simulink library "honestlibrary"  (R2013b)
settings: Solver=ode45  StartTime=0.0  StopTime=10.0  RelTol=1e-3
libraries: honestlibrary x192, xbsIndex_r4 x32
(part 1 of 2)
settings Model: Creator=sergio  LastModifiedBy=root

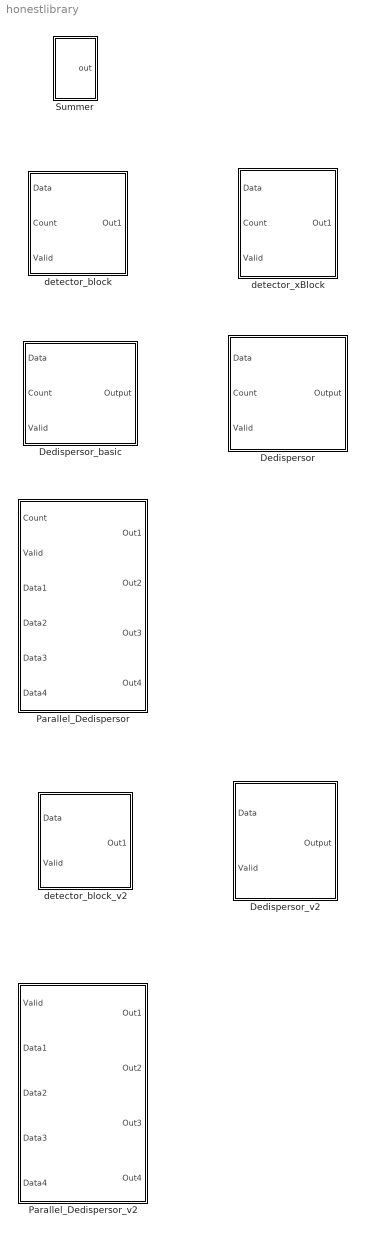
== system honestlibrary ==
  Dedispersor : Subsystem  mask(Detector de FRB (hasta 1024 canales)){DM_Vector=[0:1:15]}
      mask prompts: DM_Vector "DM Vector"
      mask help: Recibe un vector de DM asociado al retardo de cada canal y genera bloques detectores básicos para dedispersar la señal entregada.
      mask init:
      | config.source = str2func('honest_detectorv2');
      | config.toplevel = gcb;
      | config.depend = {'honest_detectorv2.m'};
      | xBlock(config, {DM_Vector});
  Dedispersor_basic : Subsystem  mask(Detector de FRB (hasta 31 canales)){DM_Vector=[0:1:31]}
      mask prompts: DM_Vector "DM Vector"
      mask help: Recibe un vector de DM asociado al retardo de cada canal y genera bloques detectores básicos para dedispersar la señal entregada.
      mask init:
      | config.source = str2func('honest_detector');
      | config.toplevel = gcb;
      | config.depend = {'honest_detector.m'};
      | xBlock(config, {DM_Vector});
  Dedispersor_v2 : Subsystem  mask(Detector de FRB (hasta 1024 canales)){DM_Vector=[0:1:15]}
      mask prompts: DM_Vector "DM Vector"
      mask help:
      | Recibe un vector de DM asociado al retardo de cada canal y genera bloques detectores básicos para dedispersar la señal entregada.
      | Esta versión incorpora un contador de nbits en cada bloque de dedispersión.
      mask init:
      | config.source = str2func('honest_detector_v2');
      | config.toplevel = gcb;
      | config.depend = {'honest_detector_v2.m'};
      | xBlock(config, {DM_Vector});
  Parallel_Dedispersor : Subsystem  mask(Parallel Dedispersor){n_inputs=4, DM_Vector=[1:1:64]}
      mask prompts: n_inputs "Number of Inputs"; DM_Vector "DM Vector"
      mask help:
      | Parallel dedispersor takes two parameters:
      |
      | - DM Vector
      | - Number of Inputs
      |
      | Then dedisperses the incoming serial or n-bus channels according to the DM Vector format. Each input can handle 1023 different channels.
      mask init:
      | honest_parallel_detector_init(gcb,'n_inputs',n_inputs,'DM_Vector',DM_Vector);
      settings: AttributesFormatString=Inputs: 4, Channels: 64
  Parallel_Dedispersor_v2 : Subsystem  mask(Parallel Dedispersor v2){DM_Vector=[1:1:64], n_inputs=4}
      mask prompts: DM_Vector "DM Vector"; n_inputs "Number of Inputs"
      mask help:
      | Parallel dedispersor (v2) takes three parameters:
      |
      | - DM Vector
      | - Number of Inputs
      | - Number of Bits (Counter)
      |
      | Then dedisperses the incoming serial or n-bus channels according to the DM Vector format. Each input can handle 1023 different channels.
      | Each detector block contains a counter activated by the valid signal.
      mask init:
      | honest_parallel_detector_init_v2(gcb,'n_inputs',n_inputs,'DM_Vector',DM_Vector)
      settings: AttributesFormatString=Inputs: 4, Channels: 64
  Summer : Subsystem  mask(summer){num1=1, num2=1}
      mask prompts: num1 "Number 1"; num2 "Number 2"
      mask help: It adds things
      mask init:
      | summer_init(gcb,'num1',num1,'num2',num2);
      settings: AttributesFormatString=1,1
      mask Help: (you can add HTML here to make ir more beauty)
  detector_block : Subsystem  mask(Basic block for FRB detection){chn=3, lat=3}
      mask prompts: chn "Channel"; lat "Latency"
      mask help: Delays a certain channel a number of latency clock cycles, according to the fixed DM table.
      mask init:
      | detector_block_init(gcb,'chn',chn,'lat',lat)
      settings: AttributesFormatString=3,3
      mask Display:
      | port_label ('input',1,'Data')
      | port_label ('input',2,'Count')
      | port_label ('input',3,'En')
      | port_label ('output',1,'Out')
  detector_block_v2 : Subsystem  mask(Basic block for FRB detection){chn=4, lat=9, nbits=2}
      mask prompts: chn "Channel"; lat "Latency"; nbits "Number of Bits (Counter)"
      mask help:
      | Delays a certain channel a number of latency clock cycles, according to the fixed DM table.
      | This version incorporates an internal counter (nbits) to know when store or give a certain value.
      mask init:
      | detector_block_init_v2(gcb,'chn',chn,'lat',lat,'nbits',nbits)
      settings: AttributesFormatString=Channel: 4, Delay: 9
  detector_xBlock : Subsystem  RequirementInfo="{}  %GIDa_91708f24_1105_4a04_a381_067cf6e93763"  mask(Basic block for FRB detection){channel=2, latency=9}
      mask prompts: channel "Channel Number"
      mask help: Delays a certain channel a number of latency clock cycles, according to a fixed DM table.
      mask init:
      | config.source = str2func('detector_xblock');
      | config.toplevel = gcb;
      | config.depend = {'detector_xblock.m'};
      | xBlock(config, {channel, latency});
      | set_param(gcb, 'AttributesFormatString',[num2str(channel),',',num2str(latency)])
      settings: AttributesFormatString=2,9

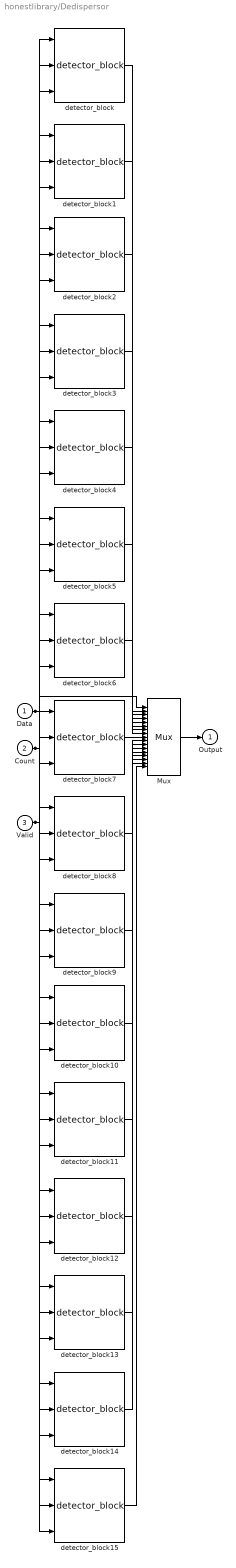
== system honestlibrary/Dedispersor ==
  Data : Inport
  Count : Inport  Port=2
  Valid : Inport  Port=3
  Mux : xbsIndex_r4/Mux  inputs=16  en=off  latency=0  precision=Full  arith_type=Unsigned  n_bits=16  bin_pt=14  quantization=Truncate  overflow=Wrap  dbl_ovrd=off  block_type=mux
  detector_block : honestlibrary/detector_block  chn=0  lat=1
      settings: AttributesFormatString=3,3
  detector_block1 : honestlibrary/detector_block  chn=1  lat=2
      settings: AttributesFormatString=3,3
  detector_block10 : honestlibrary/detector_block  chn=10  lat=11
      settings: AttributesFormatString=3,3
  detector_block11 : honestlibrary/detector_block  chn=11  lat=12
      settings: AttributesFormatString=3,3
  detector_block12 : honestlibrary/detector_block  chn=12  lat=13
      settings: AttributesFormatString=3,3
  detector_block13 : honestlibrary/detector_block  chn=13  lat=14
      settings: AttributesFormatString=3,3
  detector_block14 : honestlibrary/detector_block  chn=14  lat=15
      settings: AttributesFormatString=3,3
  detector_block15 : honestlibrary/detector_block  chn=15  lat=16
      settings: AttributesFormatString=3,3
  detector_block2 : honestlibrary/detector_block  chn=2  lat=3
      settings: AttributesFormatString=3,3
  detector_block3 : honestlibrary/detector_block  chn=3  lat=4
      settings: AttributesFormatString=3,3
  detector_block4 : honestlibrary/detector_block  chn=4  lat=5
      settings: AttributesFormatString=3,3
  detector_block5 : honestlibrary/detector_block  chn=5  lat=6
      settings: AttributesFormatString=3,3
  detector_block6 : honestlibrary/detector_block  chn=6  lat=7
      settings: AttributesFormatString=3,3
  detector_block7 : honestlibrary/detector_block  chn=7  lat=8
      settings: AttributesFormatString=3,3
  detector_block8 : honestlibrary/detector_block  chn=8  lat=9
      settings: AttributesFormatString=3,3
  detector_block9 : honestlibrary/detector_block  chn=9  lat=10
      settings: AttributesFormatString=3,3
  Output : Outport
  wires:
  Data/1 -> detector_block15/1, detector_block14/1, detector_block13/1, detector_block12/1, detector_block11/1, detector_block10/1, detector_block9/1, detector_block8/1, detector_block7/1, detector_block6/1, detector_block5/1, detector_block4/1, detector_block3/1, detector_block2/1, detector_block1/1, detector_block/1
  Count/1 -> Mux/1, detector_block15/2, detector_block14/2, detector_block13/2, detector_block12/2, detector_block11/2, detector_block10/2, detector_block9/2, detector_block8/2, detector_block7/2, detector_block6/2, detector_block5/2, detector_block4/2, detector_block3/2, detector_block2/2, detector_block1/2, detector_block/2
  Valid/1 -> detector_block15/3, detector_block14/3, detector_block13/3, detector_block12/3, detector_block11/3, detector_block10/3, detector_block9/3, detector_block8/3, detector_block7/3, detector_block6/3, detector_block5/3, detector_block4/3, detector_block3/3, detector_block2/3, detector_block1/3, detector_block/3
  Mux/1 -> Output/1
  detector_block15/1 -> Mux/17
  detector_block14/1 -> Mux/16
  detector_block13/1 -> Mux/15
  detector_block12/1 -> Mux/14
  detector_block11/1 -> Mux/13
  detector_block10/1 -> Mux/12
  detector_block9/1 -> Mux/11
  detector_block8/1 -> Mux/10
  detector_block7/1 -> Mux/9
  detector_block6/1 -> Mux/8
  detector_block5/1 -> Mux/7
  detector_block4/1 -> Mux/6
  detector_block3/1 -> Mux/5
  detector_block2/1 -> Mux/4
  detector_block1/1 -> Mux/3
  detector_block/1 -> Mux/2

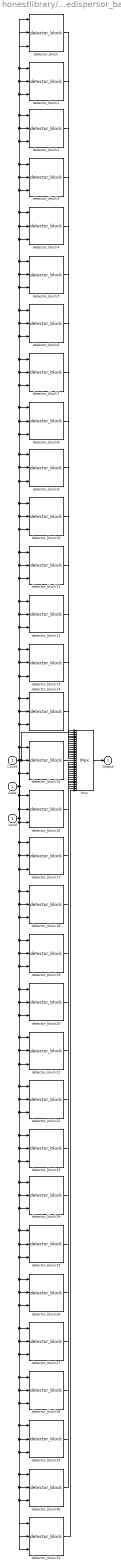
== system honestlibrary/Dedispersor_basic ==
  Data : Inport
  Count : Inport  Port=2
  Valid : Inport  Port=3
  Mux : xbsIndex_r4/Mux  inputs=32  en=off  latency=0  precision=Full  arith_type=Unsigned  n_bits=16  bin_pt=14  quantization=Truncate  overflow=Wrap  dbl_ovrd=off  block_type=mux
  detector_block : honestlibrary/detector_block  chn=0  lat=1
      settings: AttributesFormatString=3,3
  detector_block1 : honestlibrary/detector_block  chn=1  lat=2
      settings: AttributesFormatString=3,3
  detector_block10 : honestlibrary/detector_block  chn=10  lat=11
      settings: AttributesFormatString=3,3
  detector_block11 : honestlibrary/detector_block  chn=11  lat=12
      settings: AttributesFormatString=3,3
  detector_block12 : honestlibrary/detector_block  chn=12  lat=13
      settings: AttributesFormatString=3,3
  detector_block13 : honestlibrary/detector_block  chn=13  lat=14
      settings: AttributesFormatString=3,3
  detector_block14 : honestlibrary/detector_block  chn=14  lat=15
      settings: AttributesFormatString=3,3
  detector_block15 : honestlibrary/detector_block  chn=15  lat=16
      settings: AttributesFormatString=3,3
  detector_block16 : honestlibrary/detector_block  chn=16  lat=17
      settings: AttributesFormatString=3,3
  detector_block17 : honestlibrary/detector_block  chn=17  lat=18
      settings: AttributesFormatString=3,3
  detector_block18 : honestlibrary/detector_block  chn=18  lat=19
      settings: AttributesFormatString=3,3
  detector_block19 : honestlibrary/detector_block  chn=19  lat=20
      settings: AttributesFormatString=3,3
  detector_block2 : honestlibrary/detector_block  chn=2  lat=3
      settings: AttributesFormatString=3,3
  detector_block20 : honestlibrary/detector_block  chn=20  lat=21
      settings: AttributesFormatString=3,3
  detector_block21 : honestlibrary/detector_block  chn=21  lat=22
      settings: AttributesFormatString=3,3
  detector_block22 : honestlibrary/detector_block  chn=22  lat=23
      settings: AttributesFormatString=3,3
  detector_block23 : honestlibrary/detector_block  chn=23  lat=24
      settings: AttributesFormatString=3,3
  detector_block24 : honestlibrary/detector_block  chn=24  lat=25
      settings: AttributesFormatString=3,3
  detector_block25 : honestlibrary/detector_block  chn=25  lat=26
      settings: AttributesFormatString=3,3
  detector_block26 : honestlibrary/detector_block  chn=26  lat=27
      settings: AttributesFormatString=3,3
  detector_block27 : honestlibrary/detector_block  chn=27  lat=28
      settings: AttributesFormatString=3,3
  detector_block28 : honestlibrary/detector_block  chn=28  lat=29
      settings: AttributesFormatString=3,3
  detector_block29 : honestlibrary/detector_block  chn=29  lat=30
      settings: AttributesFormatString=3,3
  detector_block3 : honestlibrary/detector_block  chn=3  lat=4
      settings: AttributesFormatString=3,3
  detector_block30 : honestlibrary/detector_block  chn=30  lat=31
      settings: AttributesFormatString=3,3
  detector_block31 : honestlibrary/detector_block  chn=31  lat=32
      settings: AttributesFormatString=3,3
  detector_block4 : honestlibrary/detector_block  chn=4  lat=5
      settings: AttributesFormatString=3,3
  detector_block5 : honestlibrary/detector_block  chn=5  lat=6
      settings: AttributesFormatString=3,3
  detector_block6 : honestlibrary/detector_block  chn=6  lat=7
      settings: AttributesFormatString=3,3
  detector_block7 : honestlibrary/detector_block  chn=7  lat=8
      settings: AttributesFormatString=3,3
  detector_block8 : honestlibrary/detector_block  chn=8  lat=9
      settings: AttributesFormatString=3,3
  detector_block9 : honestlibrary/detector_block  chn=9  lat=10
      settings: AttributesFormatString=3,3
  Output : Outport
  wires:
  Data/1 -> detector_block31/1, detector_block30/1, detector_block29/1, detector_block28/1, detector_block27/1, detector_block26/1, detector_block25/1, detector_block24/1, detector_block23/1, detector_block22/1, detector_block21/1, detector_block20/1, detector_block19/1, detector_block18/1, detector_block17/1, detector_block16/1, detector_block1/1, detector_block/1, detector_block2/1, detector_block3/1, detector_block4/1, detector_block5/1, detector_block6/1, detector_block7/1, detector_block8/1, detector_block9/1, detector_block10/1, detector_block11/1, detector_block12/1, detector_block13/1, detector_block14/1, detector_block15/1
  Count/1 -> detector_block31/2, detector_block30/2, detector_block29/2, detector_block28/2, detector_block27/2, detector_block26/2, detector_block25/2, detector_block24/2, detector_block23/2, detector_block22/2, detector_block21/2, detector_block20/2, detector_block19/2, detector_block18/2, detector_block17/2, detector_block16/2, Mux/1, detector_block15/2, detector_block1/2, detector_block/2, detector_block2/2, detector_block3/2, detector_block4/2, detector_block5/2, detector_block6/2, detector_block7/2, detector_block8/2, detector_block9/2, detector_block10/2, detector_block11/2, detector_block12/2, detector_block13/2, detector_block14/2
  Valid/1 -> detector_block31/3, detector_block30/3, detector_block29/3, detector_block28/3, detector_block27/3, detector_block26/3, detector_block25/3, detector_block24/3, detector_block23/3, detector_block22/3, detector_block21/3, detector_block20/3, detector_block19/3, detector_block18/3, detector_block17/3, detector_block16/3, detector_block1/3, detector_block/3, detector_block2/3, detector_block3/3, detector_block4/3, detector_block5/3, detector_block6/3, detector_block7/3, detector_block8/3, detector_block9/3, detector_block10/3, detector_block11/3, detector_block12/3, detector_block13/3, detector_block14/3, detector_block15/3
  Mux/1 -> Output/1
  detector_block31/1 -> Mux/33
  detector_block30/1 -> Mux/32
  detector_block29/1 -> Mux/31
  detector_block28/1 -> Mux/30
  detector_block27/1 -> Mux/29
  detector_block26/1 -> Mux/28
  detector_block25/1 -> Mux/27
  detector_block24/1 -> Mux/26
  detector_block23/1 -> Mux/25
  detector_block22/1 -> Mux/24
  detector_block21/1 -> Mux/23
  detector_block20/1 -> Mux/22
  detector_block19/1 -> Mux/21
  detector_block18/1 -> Mux/20
  detector_block17/1 -> Mux/19
  detector_block16/1 -> Mux/18
  detector_block15/1 -> Mux/17
  detector_block14/1 -> Mux/16
  detector_block13/1 -> Mux/15
  detector_block12/1 -> Mux/14
  detector_block11/1 -> Mux/13
  detector_block10/1 -> Mux/12
  detector_block9/1 -> Mux/11
  detector_block8/1 -> Mux/10
  detector_block7/1 -> Mux/9
  detector_block6/1 -> Mux/8
  detector_block5/1 -> Mux/7
  detector_block4/1 -> Mux/6
  detector_block3/1 -> Mux/5
  detector_block2/1 -> Mux/4
  detector_block1/1 -> Mux/3
  detector_block/1 -> Mux/2

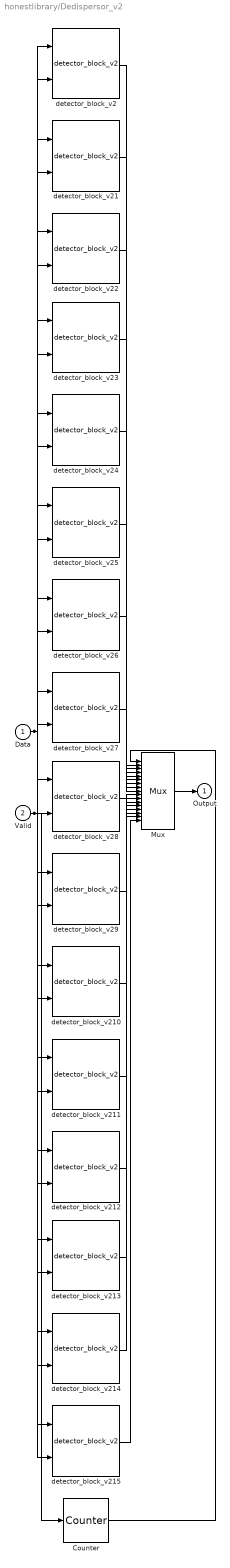
== system honestlibrary/Dedispersor_v2 ==
  Data : Inport
  Valid : Inport  Port=2
  Counter : xbsIndex_r4/Counter  cnt_type=Free Running  cnt_to=Inf  operation=Up  start_count=0  cnt_by_val=1  arith_type=Unsigned  n_bits=4  bin_pt=0  load_pin=off  rst=off  en=on  explicit_period=on  period=1  dbl_ovrd=off  use_behavioral_HDL=off  implementation=Fabric  block_type=counter
  Mux : xbsIndex_r4/Mux  inputs=16  en=off  latency=0  precision=Full  arith_type=Unsigned  n_bits=16  bin_pt=14  quantization=Truncate  overflow=Wrap  dbl_ovrd=off  block_type=mux
  detector_block_v2 : honestlibrary/detector_block_v2  chn=0  lat=1  nbits=4
      settings: AttributesFormatString=Channel: 4, Delay: 9
  detector_block_v21 : honestlibrary/detector_block_v2  chn=1  lat=2  nbits=4
      settings: AttributesFormatString=Channel: 4, Delay: 9
  detector_block_v210 : honestlibrary/detector_block_v2  chn=10  lat=11  nbits=4
      settings: AttributesFormatString=Channel: 4, Delay: 9
  detector_block_v211 : honestlibrary/detector_block_v2  chn=11  lat=12  nbits=4
      settings: AttributesFormatString=Channel: 4, Delay: 9
  detector_block_v212 : honestlibrary/detector_block_v2  chn=12  lat=13  nbits=4
      settings: AttributesFormatString=Channel: 4, Delay: 9
  detector_block_v213 : honestlibrary/detector_block_v2  chn=13  lat=14  nbits=4
      settings: AttributesFormatString=Channel: 4, Delay: 9
  detector_block_v214 : honestlibrary/detector_block_v2  chn=14  lat=15  nbits=4
      settings: AttributesFormatString=Channel: 4, Delay: 9
  detector_block_v215 : honestlibrary/detector_block_v2  chn=15  lat=16  nbits=4
      settings: AttributesFormatString=Channel: 4, Delay: 9
  detector_block_v22 : honestlibrary/detector_block_v2  chn=2  lat=3  nbits=4
      settings: AttributesFormatString=Channel: 4, Delay: 9
  detector_block_v23 : honestlibrary/detector_block_v2  chn=3  lat=4  nbits=4
      settings: AttributesFormatString=Channel: 4, Delay: 9
  detector_block_v24 : honestlibrary/detector_block_v2  chn=4  lat=5  nbits=4
      settings: AttributesFormatString=Channel: 4, Delay: 9
  detector_block_v25 : honestlibrary/detector_block_v2  chn=5  lat=6  nbits=4
      settings: AttributesFormatString=Channel: 4, Delay: 9
  detector_block_v26 : honestlibrary/detector_block_v2  chn=6  lat=7  nbits=4
      settings: AttributesFormatString=Channel: 4, Delay: 9
  detector_block_v27 : honestlibrary/detector_block_v2  chn=7  lat=8  nbits=4
      settings: AttributesFormatString=Channel: 4, Delay: 9
  detector_block_v28 : honestlibrary/detector_block_v2  chn=8  lat=9  nbits=4
      settings: AttributesFormatString=Channel: 4, Delay: 9
  detector_block_v29 : honestlibrary/detector_block_v2  chn=9  lat=10  nbits=4
      settings: AttributesFormatString=Channel: 4, Delay: 9
  Output : Outport
  wires:
  Data/1 -> detector_block_v215/1, detector_block_v214/1, detector_block_v213/1, detector_block_v212/1, detector_block_v211/1, detector_block_v210/1, detector_block_v29/1, detector_block_v28/1, detector_block_v27/1, detector_block_v26/1, detector_block_v25/1, detector_block_v24/1, detector_block_v23/1, detector_block_v22/1, detector_block_v21/1, detector_block_v2/1
  Valid/1 -> Counter/1, detector_block_v215/2, detector_block_v214/2, detector_block_v213/2, detector_block_v212/2, detector_block_v211/2, detector_block_v210/2, detector_block_v29/2, detector_block_v28/2, detector_block_v27/2, detector_block_v26/2, detector_block_v25/2, detector_block_v24/2, detector_block_v23/2, detector_block_v22/2, detector_block_v21/2, detector_block_v2/2
  Mux/1 -> Output/1
  detector_block_v215/1 -> Mux/17
  detector_block_v214/1 -> Mux/16
  detector_block_v213/1 -> Mux/15
  detector_block_v212/1 -> Mux/14
  detector_block_v211/1 -> Mux/13
  detector_block_v210/1 -> Mux/12
  detector_block_v29/1 -> Mux/11
  detector_block_v28/1 -> Mux/10
  detector_block_v27/1 -> Mux/9
  detector_block_v26/1 -> Mux/8
  detector_block_v25/1 -> Mux/7
  detector_block_v24/1 -> Mux/6
  detector_block_v23/1 -> Mux/5
  detector_block_v22/1 -> Mux/4
  detector_block_v21/1 -> Mux/3
  detector_block_v2/1 -> Mux/2
  Counter/1 -> Mux/1

== system honestlibrary/Parallel_Dedispersor ==
  Count : Inport
  Valid : Inport  Port=2
  Data1 : Inport  Port=3
  Data2 : Inport  Port=4
  Data3 : Inport  Port=5
  Data4 : Inport  Port=6
  Dedispersor1 : Subsystem  mask(Detector de FRB (hasta 1024 canales)){DM_Vector=[1 5 9 13 17 21 25 29 33 37 41 45 49 53 57 61]}
      mask prompts: DM_Vector "DM Vector"
      mask help: Recibe un vector de DM asociado al retardo de cada canal y genera bloques detectores básicos para dedispersar la señal entregada.
      mask init:
      | config.source = str2func('honest_detectorv2');
      | config.toplevel = gcb;
      | config.depend = {'honest_detectorv2.m'};
      | xBlock(config, {DM_Vector});
  Dedispersor2 : Subsystem  mask(Detector de FRB (hasta 1024 canales)){DM_Vector=[2 6 10 14 18 22 26 30 34 38 42 46 50 54 58 62]}
      mask prompts: DM_Vector "DM Vector"
      mask help: Recibe un vector de DM asociado al retardo de cada canal y genera bloques detectores básicos para dedispersar la señal entregada.
      mask init:
      | config.source = str2func('honest_detectorv2');
      | config.toplevel = gcb;
      | config.depend = {'honest_detectorv2.m'};
      | xBlock(config, {DM_Vector});
  Dedispersor3 : Subsystem  mask(Detector de FRB (hasta 1024 canales)){DM_Vector=[3 7 11 15 19 23 27 31 35 39 43 47 51 55 59 63]}
      mask prompts: DM_Vector "DM Vector"
      mask help: Recibe un vector de DM asociado al retardo de cada canal y genera bloques detectores básicos para dedispersar la señal entregada.
      mask init:
      | config.source = str2func('honest_detectorv2');
      | config.toplevel = gcb;
      | config.depend = {'honest_detectorv2.m'};
      | xBlock(config, {DM_Vector});
  Dedispersor4 : Subsystem  mask(Detector de FRB (hasta 1024 canales)){DM_Vector=[4 8 12 16 20 24 28 32 36 40 44 48 52 56 60 64]}
      mask prompts: DM_Vector "DM Vector"
      mask help: Recibe un vector de DM asociado al retardo de cada canal y genera bloques detectores básicos para dedispersar la señal entregada.
      mask init:
      | config.source = str2func('honest_detectorv2');
      | config.toplevel = gcb;
      | config.depend = {'honest_detectorv2.m'};
      | xBlock(config, {DM_Vector});
  Out1 : Outport
  Out2 : Outport  Port=2
  Out3 : Outport  Port=3
  Out4 : Outport  Port=4
  wires:
  Count/1 -> Dedispersor1/2(Count), Dedispersor2/2(Count), Dedispersor3/2(Count), Dedispersor4/2(Count)
  Valid/1 -> Dedispersor1/3(Valid), Dedispersor2/3(Valid), Dedispersor3/3(Valid), Dedispersor4/3(Valid)
  Data1/1 -> Dedispersor1/1(Data)
  Data2/1 -> Dedispersor2/1(Data)
  Data3/1 -> Dedispersor3/1(Data)
  Data4/1 -> Dedispersor4/1(Data)
  Dedispersor1/1(Output) -> Out1/1
  Dedispersor2/1(Output) -> Out2/1
  Dedispersor3/1(Output) -> Out3/1
  Dedispersor4/1(Output) -> Out4/1

== system honestlibrary/Parallel_Dedispersor_v2 ==
  Valid : Inport
  Data1 : Inport  Port=2
  Data2 : Inport  Port=3
  Data3 : Inport  Port=4
  Data4 : Inport  Port=5
  Dedispersor_v2_1 : Subsystem  mask(Detector de FRB (hasta 1024 canales)){DM_Vector=[1 5 9 13 17 21 25 29 33 37 41 45 49 53 57 61]}
      mask prompts: DM_Vector "DM Vector"
      mask help:
      | Recibe un vector de DM asociado al retardo de cada canal y genera bloques detectores básicos para dedispersar la señal entregada.
      | Esta versión incorpora un contador de nbits en cada bloque de dedispersión.
      mask init:
      | config.source = str2func('honest_detector_v2');
      | config.toplevel = gcb;
      | config.depend = {'honest_detector_v2.m'};
      | xBlock(config, {DM_Vector});
  Dedispersor_v2_2 : Subsystem  mask(Detector de FRB (hasta 1024 canales)){DM_Vector=[2 6 10 14 18 22 26 30 34 38 42 46 50 54 58 62]}
      mask prompts: DM_Vector "DM Vector"
      mask help:
      | Recibe un vector de DM asociado al retardo de cada canal y genera bloques detectores básicos para dedispersar la señal entregada.
      | Esta versión incorpora un contador de nbits en cada bloque de dedispersión.
      mask init:
      | config.source = str2func('honest_detector_v2');
      | config.toplevel = gcb;
      | config.depend = {'honest_detector_v2.m'};
      | xBlock(config, {DM_Vector});
  Dedispersor_v2_3 : Subsystem  mask(Detector de FRB (hasta 1024 canales)){DM_Vector=[3 7 11 15 19 23 27 31 35 39 43 47 51 55 59 63]}
      mask prompts: DM_Vector "DM Vector"
      mask help:
      | Recibe un vector de DM asociado al retardo de cada canal y genera bloques detectores básicos para dedispersar la señal entregada.
      | Esta versión incorpora un contador de nbits en cada bloque de dedispersión.
      mask init:
      | config.source = str2func('honest_detector_v2');
      | config.toplevel = gcb;
      | config.depend = {'honest_detector_v2.m'};
      | xBlock(config, {DM_Vector});
  Dedispersor_v2_4 : Subsystem  mask(Detector de FRB (hasta 1024 canales)){DM_Vector=[4 8 12 16 20 24 28 32 36 40 44 48 52 56 60 64]}
      mask prompts: DM_Vector "DM Vector"
      mask help:
      | Recibe un vector de DM asociado al retardo de cada canal y genera bloques detectores básicos para dedispersar la señal entregada.
      | Esta versión incorpora un contador de nbits en cada bloque de dedispersión.
      mask init:
      | config.source = str2func('honest_detector_v2');
      | config.toplevel = gcb;
      | config.depend = {'honest_detector_v2.m'};
      | xBlock(config, {DM_Vector});
  Out1 : Outport
  Out2 : Outport  Port=2
  Out3 : Outport  Port=3
  Out4 : Outport  Port=4
  wires:
  Valid/1 -> Dedispersor_v2_1/2(Valid), Dedispersor_v2_2/2(Valid), Dedispersor_v2_3/2(Valid), Dedispersor_v2_4/2(Valid)
  Data1/1 -> Dedispersor_v2_1/1(Data)
  Data2/1 -> Dedispersor_v2_2/1(Data)
  Data3/1 -> Dedispersor_v2_3/1(Data)
  Data4/1 -> Dedispersor_v2_4/1(Data)
  Dedispersor_v2_1/1(Output) -> Out1/1
  Dedispersor_v2_2/1(Output) -> Out2/1
  Dedispersor_v2_3/1(Output) -> Out3/1
  Dedispersor_v2_4/1(Output) -> Out4/1

== system honestlibrary/Summer ==
  adder : xbsIndex_r4/AddSub  mode=Addition  use_carryin=off  use_carryout=off  en=off  latency=1  precision=Full  arith_type=Unsigned  n_bits=16  bin_pt=14  quantization=Truncate  overflow=Wrap  dbl_ovrd=off  use_behavioral_HDL=off  hw_selection=Fabric  pipelined=off  block_type=addsub
  const1 : xbsIndex_r4/Constant  const=1  gui_display_data_type=Fixed-point  arith_type=Unsigned  n_bits=16  bin_pt=0  preci_type=Single  exp_width=8  frac_width=24  explicit_period=on  period=1  equ=P=C  opselect=C  inp2=PCIN>>17  opr=+  inp1=P  carry=CIN  dbl_ovrd=off  block_type=constant
  const2 : xbsIndex_r4/Constant  const=1  gui_display_data_type=Fixed-point  arith_type=Unsigned  n_bits=16  bin_pt=0  preci_type=Single  exp_width=8  frac_width=24  explicit_period=on  period=1  equ=P=C  opselect=C  inp2=PCIN>>17  opr=+  inp1=P  carry=CIN  dbl_ovrd=off  block_type=constant
  out : Outport
  wires:
  const1/1 -> adder/1
  const2/1 -> adder/2
  adder/1 -> out/1

== system honestlibrary/detector_block ==
  Data : Inport
  Count : Inport  Port=2
  Valid : Inport  Port=3
  Const1 : xbsIndex_r4/Constant  const=3  gui_display_data_type=Fixed-point  arith_type=Signed (2's comp)  n_bits=16  bin_pt=0  preci_type=Single  exp_width=8  frac_width=24  explicit_period=off  period=1  equ=P=C  opselect=C  inp2=PCIN>>17  opr=+  inp1=P  carry=CIN  dbl_ovrd=off  block_type=constant
  Delay1 : xbsIndex_r4/Delay  rst=off  infoeditControl=Selection of Reset will increase slice count due to use of real FFs and instead of SRLs  en=on  latency=3  dbl_ovrd=off  reg_retiming=off  block_type=delay
  Expression1 : xbsIndex_r4/Expression  expression=a & b  align_bp=on  en=off  latency=0  precision=Full  arith_type=Unsigned  n_bits=16  bin_pt=0  dbl_ovrd=off  block_type=expr
  Relational1 : xbsIndex_r4/Relational  mode=a=b  en=off  latency=0  dbl_ovrd=off  block_type=relational
  Out1 : Outport
  wires:
  Count/1 -> Relational1/1
  Const1/1 -> Relational1/2
  Relational1/1 -> Expression1/1
  Valid/1 -> Expression1/2
  Data/1 -> Delay1/1
  Expression1/1 -> Delay1/2
  Delay1/1 -> Out1/1

== system honestlibrary/detector_block_v2 ==
  Data : Inport
  Valid : Inport  Port=2
  Const1 : xbsIndex_r4/Constant  const=4  gui_display_data_type=Fixed-point  arith_type=Signed (2's comp)  n_bits=16  bin_pt=0  preci_type=Single  exp_width=8  frac_width=24  explicit_period=off  period=1  equ=P=C  opselect=C  inp2=PCIN>>17  opr=+  inp1=P  carry=CIN  dbl_ovrd=off  block_type=constant
  Counter1 : xbsIndex_r4/Counter  cnt_type=Free Running  cnt_to=Inf  operation=Up  start_count=0  cnt_by_val=1  arith_type=Unsigned  n_bits=2  bin_pt=0  load_pin=off  rst=off  en=on  explicit_period=on  period=1  dbl_ovrd=off  use_behavioral_HDL=off  implementation=Fabric  block_type=counter
  Delay1 : xbsIndex_r4/Delay  rst=off  infoeditControl=Selection of Reset will increase slice count due to use of real FFs and instead of SRLs  en=on  latency=9  dbl_ovrd=off  reg_retiming=off  block_type=delay
  Expression1 : xbsIndex_r4/Expression  expression=a & b  align_bp=on  en=off  latency=0  precision=Full  arith_type=Unsigned  n_bits=16  bin_pt=0  dbl_ovrd=off  block_type=expr
  Relational1 : xbsIndex_r4/Relational  mode=a=b  en=off  latency=0  dbl_ovrd=off  block_type=relational
  Out1 : Outport
  wires:
  Valid/1 -> Counter1/1, Expression1/2
  Counter1/1 -> Relational1/1
  Const1/1 -> Relational1/2
  Relational1/1 -> Expression1/1
  Data/1 -> Delay1/1
  Expression1/1 -> Delay1/2
  Delay1/1 -> Out1/1

== system honestlibrary/detector_xBlock ==
  Data : Inport
  Count : Inport  Port=2
  Valid : Inport  Port=3
  Constant : xbsIndex_r4/Constant  const=2  gui_display_data_type=Fixed-point  arith_type=Unsigned  n_bits=16  bin_pt=0  preci_type=Single  exp_width=8  frac_width=24  explicit_period=off  period=1  equ=P=C  opselect=C  inp2=PCIN>>17  opr=+  inp1=P  carry=CIN  dbl_ovrd=off  block_type=constant
  Delay : xbsIndex_r4/Delay  rst=off  infoeditControl=Selection of Reset will increase slice count due to use of real FFs and instead of SRLs  en=on  latency=9  dbl_ovrd=off  reg_retiming=off  block_type=delay
  Expression : xbsIndex_r4/Expression  expression=a & b  align_bp=on  en=off  latency=0  precision=Full  arith_type=Unsigned  n_bits=16  bin_pt=0  dbl_ovrd=off  block_type=expr
  Relational : xbsIndex_r4/Relational  mode=a=b  en=off  latency=0  dbl_ovrd=off  block_type=relational
  Out1 : Outport
  wires:
  Delay/1 -> Out1/1
  Expression/1 -> Delay/2
  Data/1 -> Delay/1
  Valid/1 -> Expression/2
  Relational/1 -> Expression/1
  Constant/1 -> Relational/2
  Count/1 -> Relational/1

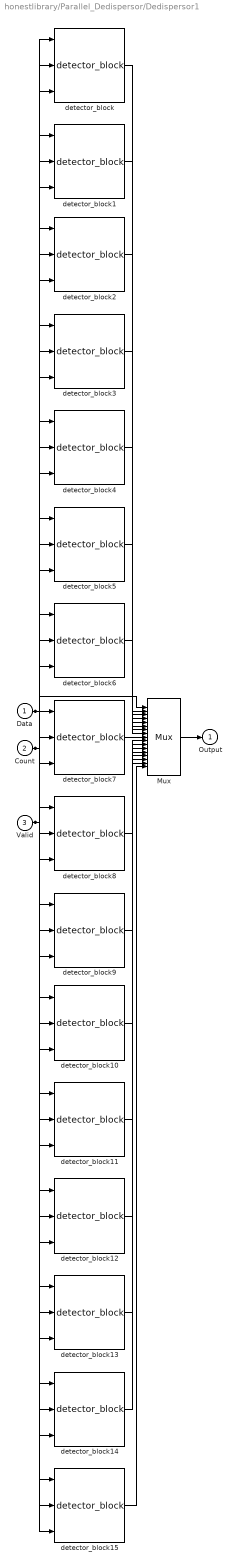
== system honestlibrary/Parallel_Dedispersor/Dedispersor1 ==
  Data : Inport
  Count : Inport  Port=2
  Valid : Inport  Port=3
  Mux : xbsIndex_r4/Mux  inputs=16  en=off  latency=0  precision=Full  arith_type=Unsigned  n_bits=16  bin_pt=14  quantization=Truncate  overflow=Wrap  dbl_ovrd=off  block_type=mux
  detector_block : honestlibrary/detector_block  chn=0  lat=1
      settings: AttributesFormatString=3,3
  detector_block1 : honestlibrary/detector_block  chn=1  lat=2
      settings: AttributesFormatString=3,3
  detector_block10 : honestlibrary/detector_block  chn=10  lat=11
      settings: AttributesFormatString=3,3
  detector_block11 : honestlibrary/detector_block  chn=11  lat=12
      settings: AttributesFormatString=3,3
  detector_block12 : honestlibrary/detector_block  chn=12  lat=13
      settings: AttributesFormatString=3,3
  detector_block13 : honestlibrary/detector_block  chn=13  lat=14
      settings: AttributesFormatString=3,3
  detector_block14 : honestlibrary/detector_block  chn=14  lat=15
      settings: AttributesFormatString=3,3
  detector_block15 : honestlibrary/detector_block  chn=15  lat=16
      settings: AttributesFormatString=3,3
  detector_block2 : honestlibrary/detector_block  chn=2  lat=3
      settings: AttributesFormatString=3,3
  detector_block3 : honestlibrary/detector_block  chn=3  lat=4
      settings: AttributesFormatString=3,3
  detector_block4 : honestlibrary/detector_block  chn=4  lat=5
      settings: AttributesFormatString=3,3
  detector_block5 : honestlibrary/detector_block  chn=5  lat=6
      settings: AttributesFormatString=3,3
  detector_block6 : honestlibrary/detector_block  chn=6  lat=7
      settings: AttributesFormatString=3,3
  detector_block7 : honestlibrary/detector_block  chn=7  lat=8
      settings: AttributesFormatString=3,3
  detector_block8 : honestlibrary/detector_block  chn=8  lat=9
      settings: AttributesFormatString=3,3
  detector_block9 : honestlibrary/detector_block  chn=9  lat=10
      settings: AttributesFormatString=3,3
  Output : Outport
  wires:
  detector_block/1 -> Mux/2
  detector_block1/1 -> Mux/3
  detector_block2/1 -> Mux/4
  detector_block3/1 -> Mux/5
  detector_block4/1 -> Mux/6
  detector_block5/1 -> Mux/7
  detector_block6/1 -> Mux/8
  detector_block7/1 -> Mux/9
  detector_block8/1 -> Mux/10
  detector_block9/1 -> Mux/11
  detector_block10/1 -> Mux/12
  detector_block11/1 -> Mux/13
  detector_block12/1 -> Mux/14
  detector_block13/1 -> Mux/15
  detector_block14/1 -> Mux/16
  detector_block15/1 -> Mux/17
  Mux/1 -> Output/1
  Valid/1 -> detector_block/3, detector_block1/3, detector_block2/3, detector_block3/3, detector_block4/3, detector_block5/3, detector_block6/3, detector_block7/3, detector_block8/3, detector_block9/3, detector_block10/3, detector_block11/3, detector_block12/3, detector_block13/3, detector_block14/3, detector_block15/3
  Count/1 -> detector_block/2, detector_block1/2, detector_block2/2, detector_block3/2, detector_block4/2, detector_block5/2, detector_block6/2, detector_block7/2, detector_block8/2, detector_block9/2, detector_block10/2, detector_block11/2, detector_block12/2, detector_block13/2, detector_block14/2, detector_block15/2, Mux/1
  Data/1 -> detector_block/1, detector_block1/1, detector_block2/1, detector_block3/1, detector_block4/1, detector_block5/1, detector_block6/1, detector_block7/1, detector_block8/1, detector_block9/1, detector_block10/1, detector_block11/1, detector_block12/1, detector_block13/1, detector_block14/1, detector_block15/1

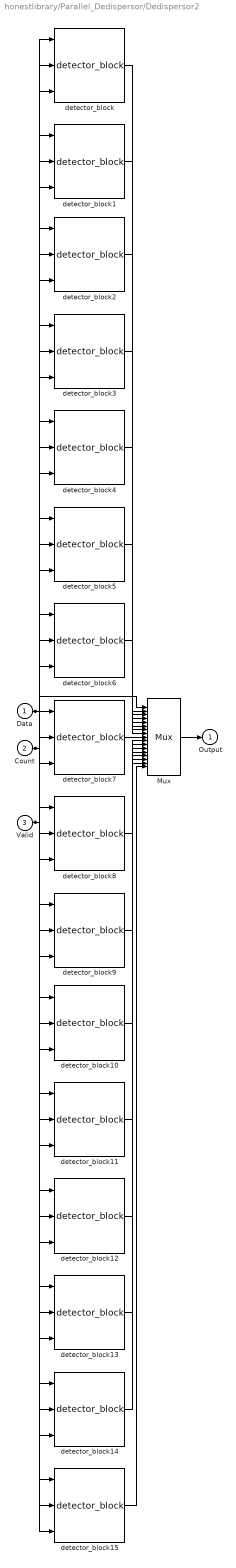
== system honestlibrary/Parallel_Dedispersor/Dedispersor2 ==
  Data : Inport
  Count : Inport  Port=2
  Valid : Inport  Port=3
  Mux : xbsIndex_r4/Mux  inputs=16  en=off  latency=0  precision=Full  arith_type=Unsigned  n_bits=16  bin_pt=14  quantization=Truncate  overflow=Wrap  dbl_ovrd=off  block_type=mux
  detector_block : honestlibrary/detector_block  chn=0  lat=1
      settings: AttributesFormatString=3,3
  detector_block1 : honestlibrary/detector_block  chn=1  lat=2
      settings: AttributesFormatString=3,3
  detector_block10 : honestlibrary/detector_block  chn=10  lat=11
      settings: AttributesFormatString=3,3
  detector_block11 : honestlibrary/detector_block  chn=11  lat=12
      settings: AttributesFormatString=3,3
  detector_block12 : honestlibrary/detector_block  chn=12  lat=13
      settings: AttributesFormatString=3,3
  detector_block13 : honestlibrary/detector_block  chn=13  lat=14
      settings: AttributesFormatString=3,3
  detector_block14 : honestlibrary/detector_block  chn=14  lat=15
      settings: AttributesFormatString=3,3
  detector_block15 : honestlibrary/detector_block  chn=15  lat=16
      settings: AttributesFormatString=3,3
  detector_block2 : honestlibrary/detector_block  chn=2  lat=3
      settings: AttributesFormatString=3,3
  detector_block3 : honestlibrary/detector_block  chn=3  lat=4
      settings: AttributesFormatString=3,3
  detector_block4 : honestlibrary/detector_block  chn=4  lat=5
      settings: AttributesFormatString=3,3
  detector_block5 : honestlibrary/detector_block  chn=5  lat=6
      settings: AttributesFormatString=3,3
  detector_block6 : honestlibrary/detector_block  chn=6  lat=7
      settings: AttributesFormatString=3,3
  detector_block7 : honestlibrary/detector_block  chn=7  lat=8
      settings: AttributesFormatString=3,3
  detector_block8 : honestlibrary/detector_block  chn=8  lat=9
      settings: AttributesFormatString=3,3
  detector_block9 : honestlibrary/detector_block  chn=9  lat=10
      settings: AttributesFormatString=3,3
  Output : Outport
  wires:
  detector_block/1 -> Mux/2
  detector_block1/1 -> Mux/3
  detector_block2/1 -> Mux/4
  detector_block3/1 -> Mux/5
  detector_block4/1 -> Mux/6
  detector_block5/1 -> Mux/7
  detector_block6/1 -> Mux/8
  detector_block7/1 -> Mux/9
  detector_block8/1 -> Mux/10
  detector_block9/1 -> Mux/11
  detector_block10/1 -> Mux/12
  detector_block11/1 -> Mux/13
  detector_block12/1 -> Mux/14
  detector_block13/1 -> Mux/15
  detector_block14/1 -> Mux/16
  detector_block15/1 -> Mux/17
  Mux/1 -> Output/1
  Valid/1 -> detector_block/3, detector_block1/3, detector_block2/3, detector_block3/3, detector_block4/3, detector_block5/3, detector_block6/3, detector_block7/3, detector_block8/3, detector_block9/3, detector_block10/3, detector_block11/3, detector_block12/3, detector_block13/3, detector_block14/3, detector_block15/3
  Count/1 -> detector_block/2, detector_block1/2, detector_block2/2, detector_block3/2, detector_block4/2, detector_block5/2, detector_block6/2, detector_block7/2, detector_block8/2, detector_block9/2, detector_block10/2, detector_block11/2, detector_block12/2, detector_block13/2, detector_block14/2, detector_block15/2, Mux/1
  Data/1 -> detector_block/1, detector_block1/1, detector_block2/1, detector_block3/1, detector_block4/1, detector_block5/1, detector_block6/1, detector_block7/1, detector_block8/1, detector_block9/1, detector_block10/1, detector_block11/1, detector_block12/1, detector_block13/1, detector_block14/1, detector_block15/1

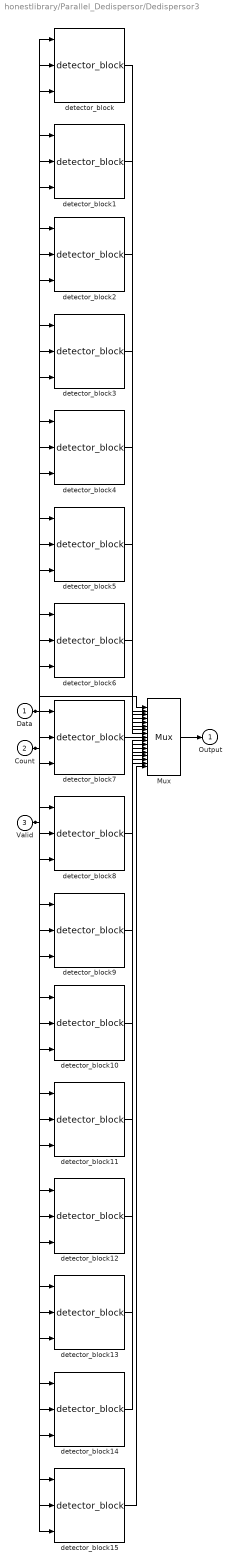
== system honestlibrary/Parallel_Dedispersor/Dedispersor3 ==
  Data : Inport
  Count : Inport  Port=2
  Valid : Inport  Port=3
  Mux : xbsIndex_r4/Mux  inputs=16  en=off  latency=0  precision=Full  arith_type=Unsigned  n_bits=16  bin_pt=14  quantization=Truncate  overflow=Wrap  dbl_ovrd=off  block_type=mux
  detector_block : honestlibrary/detector_block  chn=0  lat=1
      settings: AttributesFormatString=3,3
  detector_block1 : honestlibrary/detector_block  chn=1  lat=2
      settings: AttributesFormatString=3,3
  detector_block10 : honestlibrary/detector_block  chn=10  lat=11
      settings: AttributesFormatString=3,3
  detector_block11 : honestlibrary/detector_block  chn=11  lat=12
      settings: AttributesFormatString=3,3
  detector_block12 : honestlibrary/detector_block  chn=12  lat=13
      settings: AttributesFormatString=3,3
  detector_block13 : honestlibrary/detector_block  chn=13  lat=14
      settings: AttributesFormatString=3,3
  detector_block14 : honestlibrary/detector_block  chn=14  lat=15
      settings: AttributesFormatString=3,3
  detector_block15 : honestlibrary/detector_block  chn=15  lat=16
      settings: AttributesFormatString=3,3
  detector_block2 : honestlibrary/detector_block  chn=2  lat=3
      settings: AttributesFormatString=3,3
  detector_block3 : honestlibrary/detector_block  chn=3  lat=4
      settings: AttributesFormatString=3,3
  detector_block4 : honestlibrary/detector_block  chn=4  lat=5
      settings: AttributesFormatString=3,3
  detector_block5 : honestlibrary/detector_block  chn=5  lat=6
      settings: AttributesFormatString=3,3
  detector_block6 : honestlibrary/detector_block  chn=6  lat=7
      settings: AttributesFormatString=3,3
  detector_block7 : honestlibrary/detector_block  chn=7  lat=8
      settings: AttributesFormatString=3,3
  detector_block8 : honestlibrary/detector_block  chn=8  lat=9
      settings: AttributesFormatString=3,3
  detector_block9 : honestlibrary/detector_block  chn=9  lat=10
      settings: AttributesFormatString=3,3
  Output : Outport
  wires:
  detector_block/1 -> Mux/2
  detector_block1/1 -> Mux/3
  detector_block2/1 -> Mux/4
  detector_block3/1 -> Mux/5
  detector_block4/1 -> Mux/6
  detector_block5/1 -> Mux/7
  detector_block6/1 -> Mux/8
  detector_block7/1 -> Mux/9
  detector_block8/1 -> Mux/10
  detector_block9/1 -> Mux/11
  detector_block10/1 -> Mux/12
  detector_block11/1 -> Mux/13
  detector_block12/1 -> Mux/14
  detector_block13/1 -> Mux/15
  detector_block14/1 -> Mux/16
  detector_block15/1 -> Mux/17
  Mux/1 -> Output/1
  Valid/1 -> detector_block/3, detector_block1/3, detector_block2/3, detector_block3/3, detector_block4/3, detector_block5/3, detector_block6/3, detector_block7/3, detector_block8/3, detector_block9/3, detector_block10/3, detector_block11/3, detector_block12/3, detector_block13/3, detector_block14/3, detector_block15/3
  Count/1 -> detector_block/2, detector_block1/2, detector_block2/2, detector_block3/2, detector_block4/2, detector_block5/2, detector_block6/2, detector_block7/2, detector_block8/2, detector_block9/2, detector_block10/2, detector_block11/2, detector_block12/2, detector_block13/2, detector_block14/2, detector_block15/2, Mux/1
  Data/1 -> detector_block/1, detector_block1/1, detector_block2/1, detector_block3/1, detector_block4/1, detector_block5/1, detector_block6/1, detector_block7/1, detector_block8/1, detector_block9/1, detector_block10/1, detector_block11/1, detector_block12/1, detector_block13/1, detector_block14/1, detector_block15/1

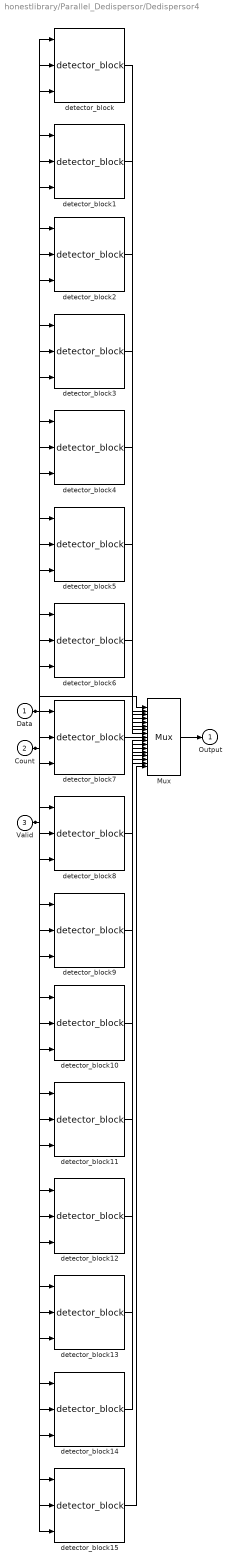
== system honestlibrary/Parallel_Dedispersor/Dedispersor4 ==
  Data : Inport
  Count : Inport  Port=2
  Valid : Inport  Port=3
  Mux : xbsIndex_r4/Mux  inputs=16  en=off  latency=0  precision=Full  arith_type=Unsigned  n_bits=16  bin_pt=14  quantization=Truncate  overflow=Wrap  dbl_ovrd=off  block_type=mux
  detector_block : honestlibrary/detector_block  chn=0  lat=1
      settings: AttributesFormatString=3,3
  detector_block1 : honestlibrary/detector_block  chn=1  lat=2
      settings: AttributesFormatString=3,3
  detector_block10 : honestlibrary/detector_block  chn=10  lat=11
      settings: AttributesFormatString=3,3
  detector_block11 : honestlibrary/detector_block  chn=11  lat=12
      settings: AttributesFormatString=3,3
  detector_block12 : honestlibrary/detector_block  chn=12  lat=13
      settings: AttributesFormatString=3,3
  detector_block13 : honestlibrary/detector_block  chn=13  lat=14
      settings: AttributesFormatString=3,3
  detector_block14 : honestlibrary/detector_block  chn=14  lat=15
      settings: AttributesFormatString=3,3
  detector_block15 : honestlibrary/detector_block  chn=15  lat=16
      settings: AttributesFormatString=3,3
  detector_block2 : honestlibrary/detector_block  chn=2  lat=3
      settings: AttributesFormatString=3,3
  detector_block3 : honestlibrary/detector_block  chn=3  lat=4
      settings: AttributesFormatString=3,3
  detector_block4 : honestlibrary/detector_block  chn=4  lat=5
      settings: AttributesFormatString=3,3
  detector_block5 : honestlibrary/detector_block  chn=5  lat=6
      settings: AttributesFormatString=3,3
  detector_block6 : honestlibrary/detector_block  chn=6  lat=7
      settings: AttributesFormatString=3,3
  detector_block7 : honestlibrary/detector_block  chn=7  lat=8
      settings: AttributesFormatString=3,3
  detector_block8 : honestlibrary/detector_block  chn=8  lat=9
      settings: AttributesFormatString=3,3
  detector_block9 : honestlibrary/detector_block  chn=9  lat=10
      settings: AttributesFormatString=3,3
  Output : Outport
  wires:
  detector_block/1 -> Mux/2
  detector_block1/1 -> Mux/3
  detector_block2/1 -> Mux/4
  detector_block3/1 -> Mux/5
  detector_block4/1 -> Mux/6
  detector_block5/1 -> Mux/7
  detector_block6/1 -> Mux/8
  detector_block7/1 -> Mux/9
  detector_block8/1 -> Mux/10
  detector_block9/1 -> Mux/11
  detector_block10/1 -> Mux/12
  detector_block11/1 -> Mux/13
  detector_block12/1 -> Mux/14
  detector_block13/1 -> Mux/15
  detector_block14/1 -> Mux/16
  detector_block15/1 -> Mux/17
  Mux/1 -> Output/1
  Valid/1 -> detector_block/3, detector_block1/3, detector_block2/3, detector_block3/3, detector_block4/3, detector_block5/3, detector_block6/3, detector_block7/3, detector_block8/3, detector_block9/3, detector_block10/3, detector_block11/3, detector_block12/3, detector_block13/3, detector_block14/3, detector_block15/3
  Count/1 -> detector_block/2, detector_block1/2, detector_block2/2, detector_block3/2, detector_block4/2, detector_block5/2, detector_block6/2, detector_block7/2, detector_block8/2, detector_block9/2, detector_block10/2, detector_block11/2, detector_block12/2, detector_block13/2, detector_block14/2, detector_block15/2, Mux/1
  Data/1 -> detector_block/1, detector_block1/1, detector_block2/1, detector_block3/1, detector_block4/1, detector_block5/1, detector_block6/1, detector_block7/1, detector_block8/1, detector_block9/1, detector_block10/1, detector_block11/1, detector_block12/1, detector_block13/1, detector_block14/1, detector_block15/1

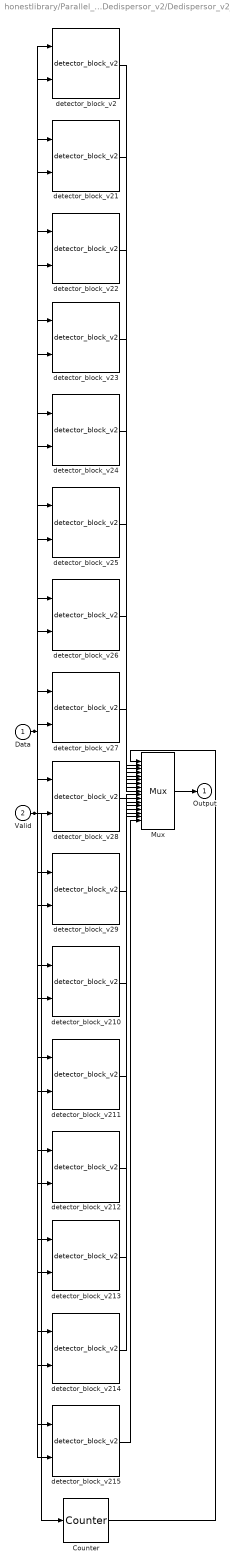
== system honestlibrary/Parallel_Dedispersor_v2/Dedispersor_v2_1 ==
  Data : Inport
  Valid : Inport  Port=2
  Counter : xbsIndex_r4/Counter  cnt_type=Free Running  cnt_to=Inf  operation=Up  start_count=0  cnt_by_val=1  arith_type=Unsigned  n_bits=4  bin_pt=0  load_pin=off  rst=off  en=on  explicit_period=on  period=1  dbl_ovrd=off  use_behavioral_HDL=off  implementation=Fabric  block_type=counter
  Mux : xbsIndex_r4/Mux  inputs=16  en=off  latency=0  precision=Full  arith_type=Unsigned  n_bits=16  bin_pt=14  quantization=Truncate  overflow=Wrap  dbl_ovrd=off  block_type=mux
  detector_block_v2 : honestlibrary/detector_block_v2  chn=0  lat=1  nbits=4
      settings: AttributesFormatString=Channel: 4, Delay: 9
  detector_block_v21 : honestlibrary/detector_block_v2  chn=1  lat=2  nbits=4
      settings: AttributesFormatString=Channel: 4, Delay: 9
  detector_block_v210 : honestlibrary/detector_block_v2  chn=10  lat=11  nbits=4
      settings: AttributesFormatString=Channel: 4, Delay: 9
  detector_block_v211 : honestlibrary/detector_block_v2  chn=11  lat=12  nbits=4
      settings: AttributesFormatString=Channel: 4, Delay: 9
  detector_block_v212 : honestlibrary/detector_block_v2  chn=12  lat=13  nbits=4
      settings: AttributesFormatString=Channel: 4, Delay: 9
  detector_block_v213 : honestlibrary/detector_block_v2  chn=13  lat=14  nbits=4
      settings: AttributesFormatString=Channel: 4, Delay: 9
  detector_block_v214 : honestlibrary/detector_block_v2  chn=14  lat=15  nbits=4
      settings: AttributesFormatString=Channel: 4, Delay: 9
  detector_block_v215 : honestlibrary/detector_block_v2  chn=15  lat=16  nbits=4
      settings: AttributesFormatString=Channel: 4, Delay: 9
  detector_block_v22 : honestlibrary/detector_block_v2  chn=2  lat=3  nbits=4
      settings: AttributesFormatString=Channel: 4, Delay: 9
  detector_block_v23 : honestlibrary/detector_block_v2  chn=3  lat=4  nbits=4
      settings: AttributesFormatString=Channel: 4, Delay: 9
  detector_block_v24 : honestlibrary/detector_block_v2  chn=4  lat=5  nbits=4
      settings: AttributesFormatString=Channel: 4, Delay: 9
  detector_block_v25 : honestlibrary/detector_block_v2  chn=5  lat=6  nbits=4
      settings: AttributesFormatString=Channel: 4, Delay: 9
  detector_block_v26 : honestlibrary/detector_block_v2  chn=6  lat=7  nbits=4
      settings: AttributesFormatString=Channel: 4, Delay: 9
  detector_block_v27 : honestlibrary/detector_block_v2  chn=7  lat=8  nbits=4
      settings: AttributesFormatString=Channel: 4, Delay: 9
  detector_block_v28 : honestlibrary/detector_block_v2  chn=8  lat=9  nbits=4
      settings: AttributesFormatString=Channel: 4, Delay: 9
  detector_block_v29 : honestlibrary/detector_block_v2  chn=9  lat=10  nbits=4
      settings: AttributesFormatString=Channel: 4, Delay: 9
  Output : Outport
  wires:
  Counter/1 -> Mux/1
  detector_block_v2/1 -> Mux/2
  detector_block_v21/1 -> Mux/3
  detector_block_v22/1 -> Mux/4
  detector_block_v23/1 -> Mux/5
  detector_block_v24/1 -> Mux/6
  detector_block_v25/1 -> Mux/7
  detector_block_v26/1 -> Mux/8
  detector_block_v27/1 -> Mux/9
  detector_block_v28/1 -> Mux/10
  detector_block_v29/1 -> Mux/11
  detector_block_v210/1 -> Mux/12
  detector_block_v211/1 -> Mux/13
  detector_block_v212/1 -> Mux/14
  detector_block_v213/1 -> Mux/15
  detector_block_v214/1 -> Mux/16
  detector_block_v215/1 -> Mux/17
  Mux/1 -> Output/1
  Valid/1 -> detector_block_v2/2, detector_block_v21/2, detector_block_v22/2, detector_block_v23/2, detector_block_v24/2, detector_block_v25/2, detector_block_v26/2, detector_block_v27/2, detector_block_v28/2, detector_block_v29/2, detector_block_v210/2, detector_block_v211/2, detector_block_v212/2, detector_block_v213/2, detector_block_v214/2, detector_block_v215/2, Counter/1
  Data/1 -> detector_block_v2/1, detector_block_v21/1, detector_block_v22/1, detector_block_v23/1, detector_block_v24/1, detector_block_v25/1, detector_block_v26/1, detector_block_v27/1, detector_block_v28/1, detector_block_v29/1, detector_block_v210/1, detector_block_v211/1, detector_block_v212/1, detector_block_v213/1, detector_block_v214/1, detector_block_v215/1
